simulink model "Simulation"  (R2016a)
settings: Solver=FixedStepAuto  StartTime=0.0  StopTime=20  FixedStep=0.01  RelTol=1e-3
undefined symbols (not defined in the file or in its folder): beta, g0, g1, g2, g3, gamma, kappa, landa, nu
(part 1 of 30)
settings Model: Creator=CAST ta 1400  LastModifiedBy=CAST ta 1400

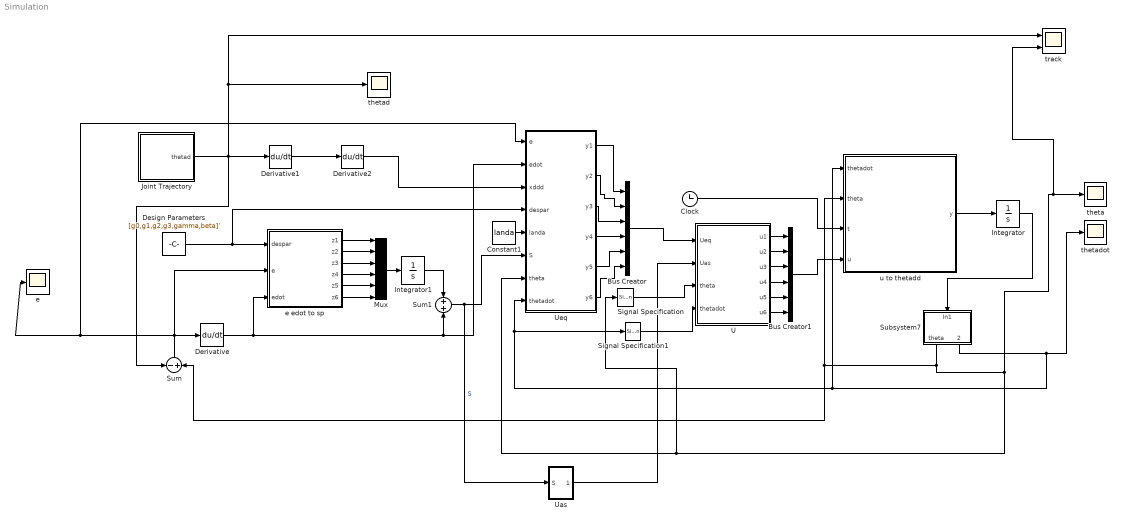
== system Simulation ==
  Bus Creator : BusCreator  Inputs=6
  Bus Creator1 : BusCreator  Inputs=6
  Clock : Clock
  Constant1 : Constant  Value=landa
  Derivative : Derivative
  Derivative1 : Derivative
  Derivative2 : Derivative
  Design Parameters : Constant  Value=[g0,g1,g2,g3,gamma,beta]'
  Integrator : Integrator  InitialCondition=[0.001*ones(6,1) ;zeros(6,1)]  LimitOutput=on  UpperSaturationLimit=10000  LowerSaturationLimit=-10000  AbsoluteTolerance=-1
  Integrator1 : Integrator  InitialCondition=[10*ones(6,1)]  UpperSaturationLimit=1000  LowerSaturationLimit=-1000  AbsoluteTolerance=-1
  Joint Trajectory : Subsystem
  Mux : Mux  Inputs=6
  Signal Specification : SignalSpecification  Dimensions=6
  Signal Specification1 : SignalSpecification  Dimensions=6
  Subsystem7 : Subsystem
  Sum : Sum  Inputs=-|+
  Sum1 : Sum  Inputs=+|+
  U : MATLAB Function  TreatAsAtomicUnit=on
  Uas : Subsystem
  Ueq : MATLAB Function  TreatAsAtomicUnit=on
  e : Scope
  e edot to sp : MATLAB Function  TreatAsAtomicUnit=on
  theta : Scope
  thetad : Scope
  thetadot : Scope
  track : Scope  NumInputPorts=2
  u to thetadd : MATLAB Function  TreatAsAtomicUnit=on
  wires:
  Sum1/1 -> Ueq/6(S), Uas/1(S)  "S"
  Derivative/1 -> Sum1/2, Ueq/2(edot), e edot to sp/3(edot)
  Clock/1 -> u to thetadd/3(t)
  Design Parameters/1 -> e edot to sp/1(despar), Ueq/4(despar)
  Joint Trajectory/1(thetad) -> Sum/1, Derivative1/1, thetad/1, track/1
  u to thetadd/1(y) -> Integrator/1
  Derivative2/1 -> Ueq/3(xddd)
  Derivative1/1 -> Derivative2/1
  Constant1/1 -> Ueq/5(landa)
  Uas/1(Uas) -> U/2(Uas)
  Ueq/1(y1) -> Bus Creator/1
  Ueq/2(y2) -> Bus Creator/2
  Ueq/3(y3) -> Bus Creator/3
  Ueq/4(y4) -> Bus Creator/4
  Ueq/5(y5) -> Bus Creator/5
  Ueq/6(y6) -> Bus Creator/6
  Bus Creator/1 -> U/1(Ueq)
  U/2(u2) -> Bus Creator1/2
  U/3(u3) -> Bus Creator1/3
  U/4(u4) -> Bus Creator1/4
  U/5(u5) -> Bus Creator1/5
  U/6(u6) -> Bus Creator1/6
  U/1(u1) -> Bus Creator1/1
  Bus Creator1/1 -> u to thetadd/4(u)
  Signal Specification1/1 -> U/4(thetadot)
  Signal Specification/1 -> U/3(theta)
  Mux/1 -> Integrator1/1
  e edot to sp/1(z1) -> Mux/1
  e edot to sp/6(z6) -> Mux/6
  Sum/1 -> e/1, Ueq/1(e), e edot to sp/2(e), Derivative/1
  e edot to sp/5(z5) -> Mux/5
  e edot to sp/4(z4) -> Mux/4
  e edot to sp/3(z3) -> Mux/3
  e edot to sp/2(z2) -> Mux/2
  Integrator1/1 -> Sum1/1
  Subsystem7/2(thetadot) -> Signal Specification1/1, Ueq/8(thetadot), u to thetadd/1(thetadot), thetadot/1
  Subsystem7/1(theta) -> track/2, theta/1, Ueq/7(theta), Signal Specification/1, Sum/2, u to thetadd/2(theta)
  Integrator/1 -> Subsystem7/1(In1)

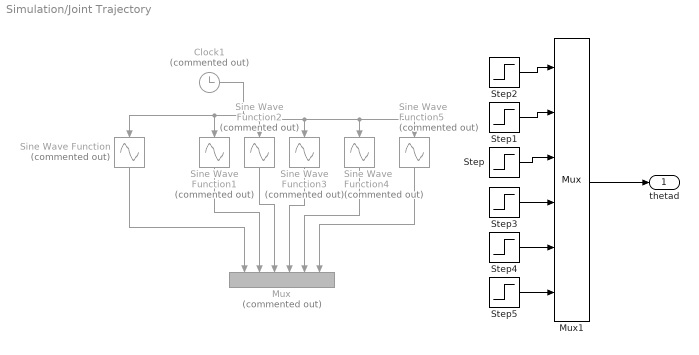
== system Simulation/Joint Trajectory ==
  Clock1 : Clock  Commented=on
  Mux : Mux  Commented=on  Inputs=6
  Mux1 : Mux  Inputs=6
  Sine Wave Function : Sin  Commented=on  TimeSource=Use external signal  Frequency=0.3  SampleTime=0
  Sine Wave Function1 : Sin  Commented=on  TimeSource=Use external signal  Frequency=0.01  SampleTime=0
  Sine Wave Function2 : Sin  Commented=on  TimeSource=Use external signal  Frequency=0.4  SampleTime=0
  Sine Wave Function3 : Sin  Commented=on  TimeSource=Use external signal  Frequency=0.01  SampleTime=0
  Sine Wave Function4 : Sin  Commented=on  TimeSource=Use external signal  Amplitude=5  Frequency=1/6  SampleTime=0
  Sine Wave Function5 : Sin  Commented=on  TimeSource=Use external signal  Amplitude=5  Bias=1  Frequency=1/5  SampleTime=0
  Step : Step  Time=0  After=-5  SampleTime=0
  Step1 : Step  Time=0  After=-5  SampleTime=0
  Step2 : Step  Time=0  After=-1  SampleTime=0
  Step3 : Step  Time=0  After=5  SampleTime=0
  Step4 : Step  Time=0  After=5  SampleTime=0
  Step5 : Step  Time=0  After=5  SampleTime=0
  thetad : Outport
  wires:
  Sine Wave Function5/1 -> Mux/6
  Sine Wave Function2/1 -> Mux/3
  Sine Wave Function4/1 -> Mux/5
  Sine Wave Function/1 -> Mux/1
  Clock1/1 -> Sine Wave Function/1, Sine Wave Function1/1, Sine Wave Function2/1, Sine Wave Function5/1, Sine Wave Function4/1, Sine Wave Function3/1
  Sine Wave Function3/1 -> Mux/4
  Sine Wave Function1/1 -> Mux/2
  Step3/1 -> Mux1/4
  Step4/1 -> Mux1/5
  Step5/1 -> Mux1/6
  Step2/1 -> Mux1/1
  Step1/1 -> Mux1/2
  Step/1 -> Mux1/3
  Mux1/1 -> thetad/1

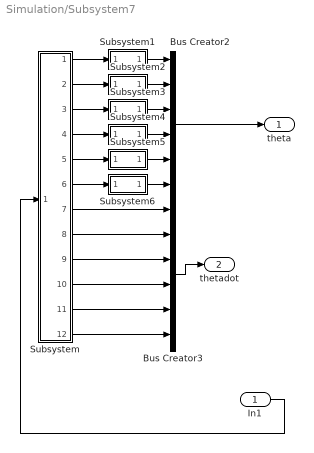
== system Simulation/Subsystem7 ==
  In1 : Inport
  Bus Creator2 : BusCreator  Inputs=6
  Bus Creator3 : BusCreator  Inputs=6
  Subsystem : Subsystem
  Subsystem1 : Subsystem
  Subsystem2 : Subsystem
  Subsystem3 : Subsystem
  Subsystem4 : Subsystem
  Subsystem5 : Subsystem
  Subsystem6 : Subsystem
  theta : Outport
  thetadot : Outport  Port=2
  wires:
  In1/1 -> Subsystem/1(In1)
  Subsystem/3(Out3) -> Subsystem3/1(In1)
  Subsystem/6(Out6) -> Subsystem6/1(In1)
  Subsystem/4(Out4) -> Subsystem4/1(In1)
  Subsystem/11(Out11) -> Bus Creator3/5
  Subsystem/1(Out1) -> Subsystem1/1(In1)
  Subsystem/9(Out9) -> Bus Creator3/3
  Subsystem/12(Out12) -> Bus Creator3/6
  Bus Creator2/1 -> theta/1
  Subsystem/5(Out5) -> Subsystem5/1(In1)
  Subsystem/10(Out10) -> Bus Creator3/4
  Subsystem/8(Out8) -> Bus Creator3/2
  Subsystem/2(Out2) -> Subsystem2/1(In1)
  Subsystem/7(Out7) -> Bus Creator3/1
  Bus Creator3/1 -> thetadot/1
  Subsystem2/1(Out1) -> Bus Creator2/2
  Subsystem1/1(Out1) -> Bus Creator2/1
  Subsystem6/1(Out1) -> Bus Creator2/6
  Subsystem3/1(Out1) -> Bus Creator2/3
  Subsystem4/1(Out1) -> Bus Creator2/4
  Subsystem5/1(Out1) -> Bus Creator2/5

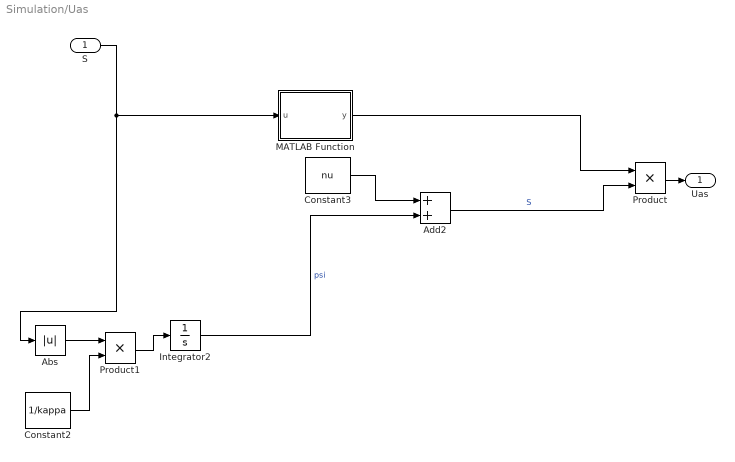
== system Simulation/Uas ==
  S : Inport
  Abs : Abs
  Add2 : Sum
  Constant2 : Constant  Value=1/kappa
  Constant3 : Constant  Value=nu
  Integrator2 : Integrator  InitialCondition=[0]
  MATLAB Function : MATLAB Function  TreatAsAtomicUnit=on
  Product : Product
  Product1 : Product
  Uas : Outport
  wires:
  Integrator2/1 -> Add2/2  "psi"
  Add2/1 -> Product/2  "S"
  Product1/1 -> Integrator2/1
  MATLAB Function/1(y) -> Product/1
  Abs/1 -> Product1/1
  S/1 -> Abs/1, MATLAB Function/1(u)
  Constant2/1 -> Product1/2
  Constant3/1 -> Add2/1
  Product/1 -> Uas/1

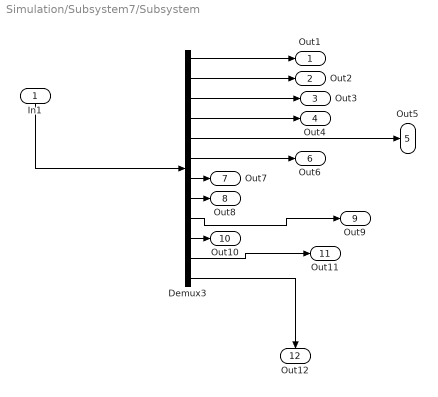
== system Simulation/Subsystem7/Subsystem ==
  In1 : Inport
  Demux3 : Demux  Outputs=12
  Out1 : Outport
  Out2 : Outport  Port=2
  Out3 : Outport  Port=3
  Out4 : Outport  Port=4
  Out5 : Outport  Port=5
  Out6 : Outport  Port=6
  Out7 : Outport  Port=7
  Out8 : Outport  Port=8
  Out9 : Outport  Port=9
  Out10 : Outport  Port=10
  Out11 : Outport  Port=11
  Out12 : Outport  Port=12
  wires:
  Demux3/1 -> Out1/1
  Demux3/9 -> Out9/1
  Demux3/10 -> Out10/1
  Demux3/7 -> Out7/1
  In1/1 -> Demux3/1
  Demux3/8 -> Out8/1
  Demux3/11 -> Out11/1
  Demux3/5 -> Out5/1
  Demux3/3 -> Out3/1
  Demux3/2 -> Out2/1
  Demux3/4 -> Out4/1
  Demux3/6 -> Out6/1
  Demux3/12 -> Out12/1

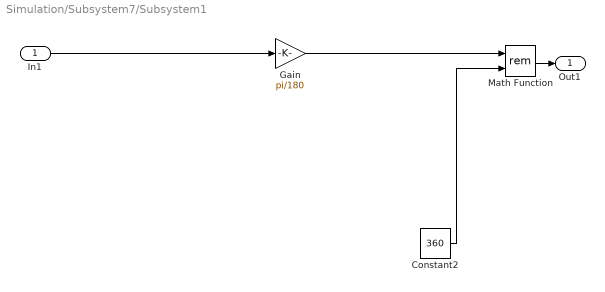
== system Simulation/Subsystem7/Subsystem1 ==
  In1 : Inport
  Constant2 : Constant  Value=360
  Gain : Gain  Gain=pi/180
  Math Function : Math  Operator=rem  SaturateOnIntegerOverflow=on
  Out1 : Outport
  wires:
  Math Function/1 -> Out1/1
  In1/1 -> Gain/1
  Constant2/1 -> Math Function/2
  Gain/1 -> Math Function/1

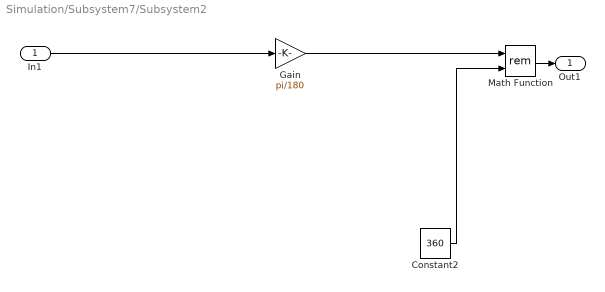
== system Simulation/Subsystem7/Subsystem2 ==
  In1 : Inport
  Constant2 : Constant  Value=360
  Gain : Gain  Gain=pi/180
  Math Function : Math  Operator=rem  SaturateOnIntegerOverflow=on
  Out1 : Outport
  wires:
  Math Function/1 -> Out1/1
  In1/1 -> Gain/1
  Constant2/1 -> Math Function/2
  Gain/1 -> Math Function/1

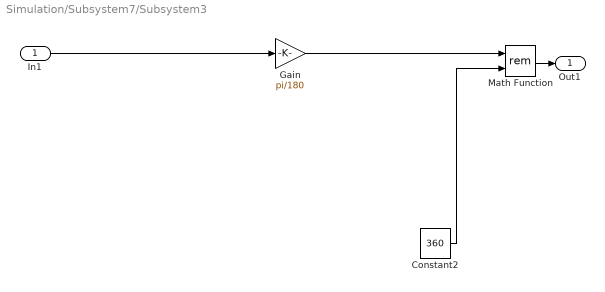
== system Simulation/Subsystem7/Subsystem3 ==
  In1 : Inport
  Constant2 : Constant  Value=360
  Gain : Gain  Gain=pi/180
  Math Function : Math  Operator=rem  SaturateOnIntegerOverflow=on
  Out1 : Outport
  wires:
  Math Function/1 -> Out1/1
  In1/1 -> Gain/1
  Constant2/1 -> Math Function/2
  Gain/1 -> Math Function/1

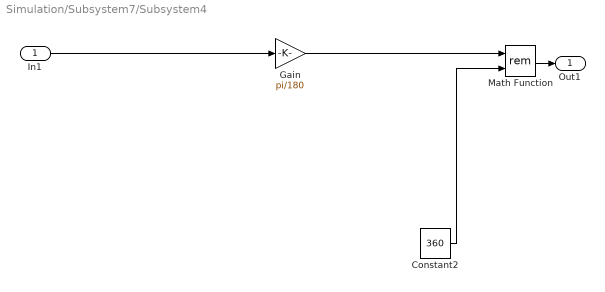
== system Simulation/Subsystem7/Subsystem4 ==
  In1 : Inport
  Constant2 : Constant  Value=360
  Gain : Gain  Gain=pi/180
  Math Function : Math  Operator=rem  SaturateOnIntegerOverflow=on
  Out1 : Outport
  wires:
  Math Function/1 -> Out1/1
  In1/1 -> Gain/1
  Constant2/1 -> Math Function/2
  Gain/1 -> Math Function/1

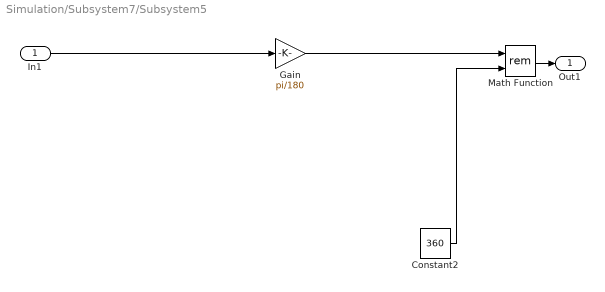
== system Simulation/Subsystem7/Subsystem5 ==
  In1 : Inport
  Constant2 : Constant  Value=360
  Gain : Gain  Gain=pi/180
  Math Function : Math  Operator=rem  SaturateOnIntegerOverflow=on
  Out1 : Outport
  wires:
  Math Function/1 -> Out1/1
  In1/1 -> Gain/1
  Constant2/1 -> Math Function/2
  Gain/1 -> Math Function/1

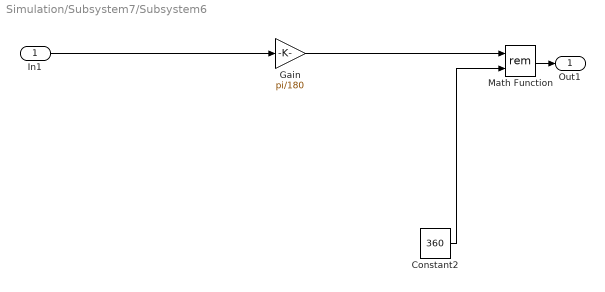
== system Simulation/Subsystem7/Subsystem6 ==
  In1 : Inport
  Constant2 : Constant  Value=360
  Gain : Gain  Gain=pi/180
  Math Function : Math  Operator=rem  SaturateOnIntegerOverflow=on
  Out1 : Outport
  wires:
  Math Function/1 -> Out1/1
  In1/1 -> Gain/1
  Constant2/1 -> Math Function/2
  Gain/1 -> Math Function/1
